simulink model "untitled"  (R2020b)
settings: Solver=VariableStepAuto  StartTime=0.0  StopTime=10.0  RelTol=1e-3
settings Model: Creator=baikp  LastModifiedBy=baikp

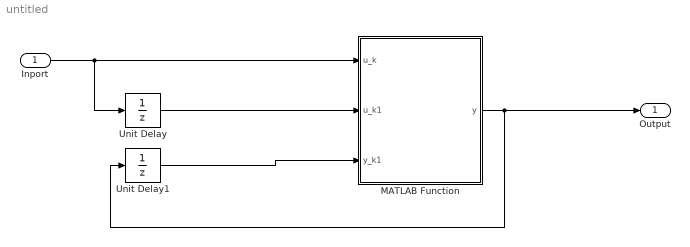
== system untitled ==
  Inport : Inport
  MATLAB Function : MATLAB Function  TreatAsAtomicUnit=on
  Unit Delay : UnitDelay  SampleTime=0.0005  HasFrameUpgradeWarning=on
  Unit Delay1 : UnitDelay  SampleTime=0.0005  HasFrameUpgradeWarning=on
  Output : Outport
  wires:
  Inport/1 -> Unit Delay/1, MATLAB Function/1(u_k)
  Unit Delay/1 -> MATLAB Function/2(u_k1)
  Unit Delay1/1 -> MATLAB Function/3(y_k1)
  MATLAB Function/1(y) -> Output/1, Unit Delay1/1

== matlab function untitled/MATLAB Function ==
  data: u_k input; y output; u_k1 input; y_k1 input
function y = fcn(u_k,u_k1,y_k1)

y = 0.8816*y_k1 + 0.05919*u_k + 0.05919*u_k1;
